simulink model "eCS_Algo_Simulation_2015b"  (R2015b)
settings: Solver=ode1  StartTime=0.0  StopTime=3  FixedStep=1/80000  RelTol=1e-3
PreLoadFcn:
  | if exist('tl_preloadfcn','file'), tl_preloadfcn(gcs,402); end
PostLoadFcn:
  | , if any(exist('dsrtsu_mdlpostloadfcn', 'file') == [2, 3, 6]), try dsrtsu_mdlpostloadfcn('Execute', bdroot); catch fprintf('Error in PostLoadFcn (dsrtsu_mdlpostloadfcn) for model "%s":\n %s\n', bdroot, lasterr); end, end,
  | if exist('tl_postloadfcn','file'), tl_postloadfcn(gcs,402); end
InitFcn:
  | Omegan=1.3024e+03;
  | xi=0.9; %0.48
  | K=0.1931;
  | K1=0.0198;
  | TauLocked=0.00255;
  | TauUnLocked=0.0042;
  | Kp=1/(2*K1);
  | Ki=Kp/((TauLocked+TauUnLocked)/2);
  | if exist('tlds_init','file'), tlds_init(gcs); end
StartFcn:
  | if exist('tlds_start','file'), tlds_start(gcs); end
StopFcn:
  | if exist('tlds_stop','file'), tlds_stop(gcs); end
model workspace (MAT data in the model file):
  au8PrevExecProfile = [0 0 0 0 0 0]
values from neighbouring files (symbols this model uses):
  AccSensor = 5    [Parameter_eCS_Algo.m]
  AlgoType = 0    [Parameter_eCS_Algo.m]
  Cxy = 1*0.017    (= 0.017)    [Acc_Init_SelV1.m]
  Cxz = 1*0.017    (= 0.017)    [Acc_Init_SelV1.m]
  Cyx = 1*0.017    (= 0.017)    [Acc_Init_SelV1.m]
  Cyz = 1*0.017    (= 0.017)    [Acc_Init_SelV1.m]
  Czx = 1*0.017    (= 0.017)    [Acc_Init_SelV1.m]
  Czy = 1*0.017    (= 0.017)    [Acc_Init_SelV1.m]
  Forced_Oscillation = 0    [Parameter_eCS_Algo.m]    (also in run_Rotation_sim.m = run)
  FreqTemperature = 10    [Acc_Init_SelV1.m]
  MaxSensorOffset = 0.3    [Acc_Init_SelV1.m]
  Mean_x_noise = 4e-3    (= 0.004)    [Acc_Init_SelV1.m]
  Mean_y_noise = 4e-3    (= 0.004)    [Acc_Init_SelV1.m]
  Mean_z_noise = 4e-3    (= 0.004)    [Acc_Init_SelV1.m]
  ODR = 8000    [Acc_Init_SelV1.m]
  offsetcorrection_on_off = 0    [Parameter_eCS_Algo.m]
  phi_pulse_rotation = 0    [Parameter_eCS_Algo.m]    (also in run_Rotation_sim.m = angle)
  pulsetype = 2    [Parameter_eCS_Algo.m]    (also in run_simulation.m = j; run_simulation_ActiveX.m = j)
  Range = 4    [Acc_Init_SelV1.m]
  sensitivity_optimisation = 0    [Parameter_eCS_Algo.m]
  TempBias = 0    [Acc_Init_SelV1.m]
  TemperatureAmp = 0    [Acc_Init_SelV1.m]
  Var_x_noise = 1.84e-9    (= 1.84e-09)    [Acc_Init_SelV1.m]
  Var_y_noise = 2.025e-09    [Acc_Init_SelV1.m]
  Var_z_noise = 1.374e-09    [Acc_Init_SelV1.m]
  w_x = 2*pi*F_x    (= 376.991118431)    [Acc_Init_SelV1.m]
  w_y = 2*pi*F_y    (= 376.991118431)    [Acc_Init_SelV1.m]
  w_z = 2*pi*F_z    (= 376.991118431)    [Acc_Init_SelV1.m]
  x_max_temp_drift = 0.061    [Acc_Init_SelV1.m]
  x_offset_enable = 0    [Acc_Init_SelV1.m]
  x_run_to_run_drift = 0.0    (= 0)    [Acc_Init_SelV1.m]
  x_temp_co_drift = 0.000    (= 0)    [Acc_Init_SelV1.m]
  Xi_x = 0.7    [Acc_Init_SelV1.m]
  Xi_y = 0.7    [Acc_Init_SelV1.m]
  Xi_z = 0.7    [Acc_Init_SelV1.m]
  y_max_temp_drift = 0.061    [Acc_Init_SelV1.m]
  y_offset_enable = 0    [Acc_Init_SelV1.m]
  y_run_to_run_drift = 0.0    (= 0)    [Acc_Init_SelV1.m]
  y_temp_co_drift = 0.000    (= 0)    [Acc_Init_SelV1.m]
  z_max_temp_drift = 0.13    [Acc_Init_SelV1.m]
  z_offset_enable = 0    [Acc_Init_SelV1.m]
  z_run_to_run_drift = 0.0    (= 0)    [Acc_Init_SelV1.m]
  z_temp_co_drift = 0.000    (= 0)    [Acc_Init_SelV1.m]
undefined symbols (not defined in the file or in its folder): controller_sample_rate, ddv, DiscIntNeverNeededParam, gmw_roada_x__m_s__, gmw_roada_y__m_s__, gmw_roadtime_2kHz, KSF_50_a_x, KSF_50_a_y, KSF_50_time, KSG_30_a_x, KSG_30_a_y, KSG_30_time, Meldorf_HindenburgstraAcceleration_x__m_s_2_, Meldorf_HindenburgstraAcceleration_y__m_s_2_, Meldorf_HindenburgstraAcceleration_z__m_s_2_, Meldorf_HindenburgstraTime__s_, pulse_FF27, pulse_MPDB, pulse_ODB40, pulse_ODB64, pulse_USNCAP, pulsetime_FF27, pulsetime_MPDB, pulsetime_ODB40, pulsetime_ODB64, pulsetime_USNCAP, Rauasphalt_60_a_x, Rauasphalt_60_a_y, Rauasphalt_60_time, sigbuilder_block, VW_416_2kHza_x_2kHz, VW_416_2kHza_y_2kHz, VW_416_2kHztime_2kHz
libraries: simulink x29, tllib x23, tl_autosar_lib x15, simulink_extras x7, LIB_TF_G_111 x2, LIB_TF_G_12_StepControl x2, LIB_TF_G_112 x1, dspsigops x1
(part 7 of 13)

== system eCS_Algo_Simulation_2015b/eCS/Subsystem/eCS/eCS/eCS_runMainFunction/BallAlgo ==
  note: [-1 : 1]
  note: [-25 ; 25]
  note: [-25 ;25]
  Pulses(x,y) : Inport
  b8IsSensitivityOpt : Inport  Port=2
  Add : Sum  Inputs=+--  mask(TL_Sum){data={'output',{'type','Int32','scaling','MperSecSqd_Algo/scIntegV_SI','show',1},'date',738573.71918759262}}
      settings: CopyFcn=if exist('tl_reset_reviewflag','file')==2,tl_reset_reviewflag(gcbh);end  DeleteFcn=if exist('delete_tlblock','file')==2,delete_tlblock(gcbh);end  NameChangeFcn=if exist('rename_tlblock','file')==2,rename_tlblock(gcbh);end  OpenFcn=if exist('tl_open_blockdlg','file')==2,tl_open_blockdlg(gcbh);else,open_system(gcbh,'parameter');end
      mask Help: eval(['if exist(''tl_online_help'',''file'') == 2, tl_online_help(''Topic'',''TL_Sum''),else, web([''jar:file:///'',matlabroot,''/help/toolbox/simulink/help.jar!/slref/' lower(get_param(gcbh,'Blocktype')) '.html''], ''-helpbrowser''),end'])
      mask Display: plot([-0.1, 1.05, NaN, -0.1, 1.05],[.01, .01, NaN, .99, .99]);
  Angle : Sum  mask(TL_Sum){data={'output',{'scaling','PowerOf2/scAngle','show',1},'date',738573.7191878357}}
      settings: AttributesFormatString=[Int16 2^-10]\n  CopyFcn=if exist('tl_reset_reviewflag','file')==2,tl_reset_reviewflag(gcbh);end  DeleteFcn=if exist('delete_tlblock','file')==2,delete_tlblock(gcbh);end  NameChangeFcn=if exist('rename_tlblock','file')==2,rename_tlblock(gcbh);end  OpenFcn=if exist('tl_open_blockdlg','file')==2,tl_open_blockdlg(gcbh);else,open_system(gcbh,'parameter');end
      mask Help: eval(['if exist(''tl_online_help'',''file'') == 2, tl_online_help(''Topic'',''TL_Sum''),else, web([''jar:file:///'',matlabroot,''/help/toolbox/simulink/help.jar!/slref/' lower(get_param(gcbh,'Blocktype')) '.html''], ''-helpbrowser''),end'])
      mask Display: plot([-0.1, 1.05, NaN, -0.1, 1.05],[.01, .01, NaN, .99, .99]);
  BallDamperSat : Saturate  UpperLimit=ddv('eCS_CFG/SI_Algo/BALL_DAMPER_SAT_MAX')  LowerLimit=ddv('eCS_CFG/SI_Algo/BALL_DAMPER_SAT_MIN')  mask(TL_Saturate){data={'output',{'type','Int32','scaling','MperSecSqd_Algo/scIntegV_SI','show',1},'lowerlimit',{'variable','eCS_CFG/SI_Algo/BALL_DAMPER_SAT_MIN'},'upperlimit',{'variable','eCS_CFG/SI_Algo/BALL_DAMPER_SAT_MAX'},'date',738573.7191880903}}
      settings: AttributesFormatString=[Int32 2^-16]\n  CopyFcn=if exist('tl_reset_reviewflag','file')==2,tl_reset_reviewflag(gcbh);end  DeleteFcn=if exist('delete_tlblock','file')==2,delete_tlblock(gcbh);end  NameChangeFcn=if exist('rename_tlblock','file')==2,rename_tlblock(gcbh);end  OpenFcn=if exist('tl_open_blockdlg','file')==2,tl_open_blockdlg(gcbh);else,open_system(gcbh,'parameter');end
      mask Help: eval(['if exist(''tl_online_help'',''file'') == 2, tl_online_help(''Topic'',''TL_Saturate''),else, web([''jar:file:///'',matlabroot,''/help/toolbox/simulink/help.jar!/slref/' lower(get_param(gcbh,'Blocktype')) '.html''], ''-helpbrowser''),end'])
      mask Display: plot([-0.1, 1.05, NaN, -0.1, 1.05],[.01, .01, NaN, .99, .99]);
  CalotteAngle1 : Gain  Gain=ddv('eCS_CFG/SI_Algo/S16_CALOTTE_ANGLE_1')  mask(TL_Gain){data={'output',{'scaling','PowerOf2/scAngle','show',1},'gain',{'variable','eCS_CFG/SI_Algo/S16_CALOTTE_ANGLE_1'},'date',738573.71918843745}}
      settings: AttributesFormatString=[Int16 2^-10]\n  CopyFcn=if exist('tl_reset_reviewflag','file')==2,tl_reset_reviewflag(gcbh);end  DeleteFcn=if exist('delete_tlblock','file')==2,delete_tlblock(gcbh);end  NameChangeFcn=if exist('rename_tlblock','file')==2,rename_tlblock(gcbh);end  OpenFcn=if exist('tl_open_blockdlg','file')==2,tl_open_blockdlg(gcbh);else,open_system(gcbh,'parameter');end
      mask Help: eval(['if exist(''tl_online_help'',''file'') == 2, tl_online_help(''Topic'',''TL_Gain''),else, web([''jar:file:///'',matlabroot,''/help/toolbox/simulink/help.jar!/slref/' lower(get_param(gcbh,'Blocktype')) '.html''], ''-helpbrowser''),end'])
      mask Display: plot([0, .88, 0],[.05, .5, .93]);
  CalotteAngle2 : Gain  Gain=ddv('eCS_CFG/SI_Algo/S16_CALOTTE_ANGLE_2')  mask(TL_Gain){data={'output',{'scaling','PowerOf2/scAngle','show',1},'gain',{'variable','eCS_CFG/SI_Algo/S16_CALOTTE_ANGLE_2'},'date',738573.71918868052}}
      settings: AttributesFormatString=[Int16 2^-10]\n  CopyFcn=if exist('tl_reset_reviewflag','file')==2,tl_reset_reviewflag(gcbh);end  DeleteFcn=if exist('delete_tlblock','file')==2,delete_tlblock(gcbh);end  NameChangeFcn=if exist('rename_tlblock','file')==2,rename_tlblock(gcbh);end  OpenFcn=if exist('tl_open_blockdlg','file')==2,tl_open_blockdlg(gcbh);else,open_system(gcbh,'parameter');end
      mask Help: eval(['if exist(''tl_online_help'',''file'') == 2, tl_online_help(''Topic'',''TL_Gain''),else, web([''jar:file:///'',matlabroot,''/help/toolbox/simulink/help.jar!/slref/' lower(get_param(gcbh,'Blocktype')) '.html''], ''-helpbrowser''),end'])
      mask Display: plot([0, .88, 0],[.05, .5, .93]);
  Cartesian To Polar : Subsystem  TreatAsAtomicUnit=on
  Demux : Demux  Outputs=2
  Function : tllib/Function  data={'stepfunctionname','ComputeBallPosition','date',738070.65144287038}  displayString=FUNCTION
  IntegSx : DiscreteIntegrator  SampleTime=-1  LimitOutput=on  UpperSaturationLimit=ddv('eCS_CFG/SI_Algo/BALL_POS_MAX')  LowerSaturationLimit=ddv('eCS_CFG/SI_Algo/BALL_POS_MIN')  ICPrevOutput=DiscIntNeverNeededParam  ICPrevScaledInput=DiscIntNeverNeededParam  mask(TL_DiscreteIntegrator){data={'logdata',{'loggingmode',1},'output',{'name','$D','scaling','MperSecSqd_Algo/scIntegS_SI','show',1},'state',{'scaling','MperSecSqd_Algo/scIntegS_SI'},'lowerlimit',{'variable','eCS_CFG/SI_Algo/BALL_POS_MIN'},'upperlimit',{'variable','eCS_CFG/SI_Algo/BALL_POS_MAX'},'date',738573.71919074073}}
      settings: AttributesFormatString=[Int16 2^-24]\n  CopyFcn=if exist('tl_reset_reviewflag') == 2, tl_reset_reviewflag(gcbh); end  DeleteFcn=if exist('delete_tlblock','file')==2,delete_tlblock(gcbh);end  NameChangeFcn=if exist('rename_tlblock','file')==2,rename_tlblock(gcbh);end  OpenFcn=if exist('tl_open_blockdlg','file')==2,tl_open_blockdlg(gcbh);else,open_system(gcbh,'parameter');end
      mask Help: eval(['if exist(''tl_online_help'',''file'') == 2, tl_online_help(''Topic'',''TL_DiscreteIntegrator''),else, web([''jar:file:///'',matlabroot,''/help/toolbox/simulink/help.jar!/slref/' lower(get_param(gcbh,'Blocktype')) '.html''], ''-helpbrowser''),end'])
      mask Display: plot([-0.1, 1.05, NaN, -0.1, 1.05],[.01, .01, NaN, .99, .99]);
  IntegSy : DiscreteIntegrator  SampleTime=-1  LimitOutput=on  UpperSaturationLimit=ddv('eCS_CFG/SI_Algo/BALL_POS_MAX')  LowerSaturationLimit=ddv('eCS_CFG/SI_Algo/BALL_POS_MIN')  ICPrevOutput=DiscIntNeverNeededParam  ICPrevScaledInput=DiscIntNeverNeededParam  mask(TL_DiscreteIntegrator){data={'logdata',{'loggingmode',1},'output',{'name','$D','scaling','MperSecSqd_Algo/scIntegS_SI','show',1},'state',{'scaling','MperSecSqd_Algo/scIntegS_SI'},'lowerlimit',{'variable','eCS_CFG/SI_Algo/BALL_POS_MIN'},'upperlimit',{'variable','eCS_CFG/SI_Algo/BALL_POS_MAX'},'date',738573.71919109952}}
      settings: AttributesFormatString=[Int16 2^-24]\n  CopyFcn=if exist('tl_reset_reviewflag') == 2, tl_reset_reviewflag(gcbh); end  DeleteFcn=if exist('delete_tlblock','file')==2,delete_tlblock(gcbh);end  NameChangeFcn=if exist('rename_tlblock','file')==2,rename_tlblock(gcbh);end  OpenFcn=if exist('tl_open_blockdlg','file')==2,tl_open_blockdlg(gcbh);else,open_system(gcbh,'parameter');end
      mask Help: eval(['if exist(''tl_online_help'',''file'') == 2, tl_online_help(''Topic'',''TL_DiscreteIntegrator''),else, web([''jar:file:///'',matlabroot,''/help/toolbox/simulink/help.jar!/slref/' lower(get_param(gcbh,'Blocktype')) '.html''], ''-helpbrowser''),end'])
      mask Display: plot([-0.1, 1.05, NaN, -0.1, 1.05],[.01, .01, NaN, .99, .99]);
  IntegVx : DiscreteIntegrator  SampleTime=-1  ICPrevOutput=DiscIntNeverNeededParam  ICPrevScaledInput=DiscIntNeverNeededParam  mask(TL_DiscreteIntegrator){data={'logdata',{'loggingmode',1},'output',{'scaling','MperSecSqd_Algo/scIntegV_SI','show',1},'state',{'scaling','MperSecSqd_Algo/scIntegV_SI'},'date',738573.71919129626}}
      settings: AttributesFormatString=[Int16 2^-16]\n  CopyFcn=if exist('tl_reset_reviewflag') == 2, tl_reset_reviewflag(gcbh); end  DeleteFcn=if exist('delete_tlblock','file')==2,delete_tlblock(gcbh);end  NameChangeFcn=if exist('rename_tlblock','file')==2,rename_tlblock(gcbh);end  OpenFcn=if exist('tl_open_blockdlg','file')==2,tl_open_blockdlg(gcbh);else,open_system(gcbh,'parameter');end
      mask Help: eval(['if exist(''tl_online_help'',''file'') == 2, tl_online_help(''Topic'',''TL_DiscreteIntegrator''),else, web([''jar:file:///'',matlabroot,''/help/toolbox/simulink/help.jar!/slref/' lower(get_param(gcbh,'Blocktype')) '.html''], ''-helpbrowser''),end'])
      mask Display: plot([-0.1, 1.05, NaN, -0.1, 1.05],[.01, .01, NaN, .99, .99]);
  IntegVy : DiscreteIntegrator  SampleTime=-1  ICPrevOutput=DiscIntNeverNeededParam  ICPrevScaledInput=DiscIntNeverNeededParam  mask(TL_DiscreteIntegrator){data={'output',{'scaling','MperSecSqd_Algo/scIntegV_SI','show',1},'state',{'scaling','MperSecSqd_Algo/scIntegV_SI'},'date',738573.71919152781}}
      settings: CopyFcn=if exist('tl_reset_reviewflag') == 2, tl_reset_reviewflag(gcbh); end  DeleteFcn=if exist('delete_tlblock','file')==2,delete_tlblock(gcbh);end  NameChangeFcn=if exist('rename_tlblock','file')==2,rename_tlblock(gcbh);end  OpenFcn=if exist('tl_open_blockdlg','file')==2,tl_open_blockdlg(gcbh);else,open_system(gcbh,'parameter');end
      mask Help: eval(['if exist(''tl_online_help'',''file'') == 2, tl_online_help(''Topic'',''TL_DiscreteIntegrator''),else, web([''jar:file:///'',matlabroot,''/help/toolbox/simulink/help.jar!/slref/' lower(get_param(gcbh,'Blocktype')) '.html''], ''-helpbrowser''),end'])
      mask Display: plot([-0.1, 1.05, NaN, -0.1, 1.05],[.01, .01, NaN, .99, .99]);
  Lut_Angle_1 : Lookup_n-D  NumberOfTableDimensions=1  BreakpointsForDimension1=ddv('eCS_CFG/SI_Algo/AU16_LUT_CALLOTE_ANGLE_1_IDX')  IndexSearchMethod=Linear search  Table=ddv('eCS_CFG/SI_Algo/AU16_LUT_CALLOTE_ANGLE_1_FACT')  ExtrapMethod=Clip  UseLastTableValue=on  InternalRulePriority=Speed  RndMeth=Simplest  InputSameDT=on  mask(TL_Lookup1D){data={'logdata',{'loggingmode',1},'input',{'variable','eCS_CFG/SI_Algo/AU16_LUT_CALLOTE_ANGLE_1_IDX'},'output',{'type','UInt16','scaling','PowerOf2/scLutY','show',1},'table',{'variable','eCS_CFG/SI_Algo/AU16_LUT_CALLOTE_ANGLE_1_FACT'},'map',{'name','CalotteAngle1_LUT','class','MERGEABLE_CONST'},'date',738573.71919193282}}
      settings: AttributesFormatString=[UInt16 2^-14]\n  CopyFcn=if exist('tl_reset_reviewflag','file')==2,tl_reset_reviewflag(gcbh);end  DeleteFcn=if exist('delete_tlblock','file')==2,delete_tlblock(gcbh);end  NameChangeFcn=if exist('rename_tlblock','file')==2,rename_tlblock(gcbh);end  OpenFcn=if exist('tl_open_blockdlg','file')==2,tl_open_blockdlg(gcbh);else,open_system(gcbh,'parameter');end
      mask Help: eval(['if exist(''tl_online_help'',''file'') == 2, tl_online_help(''Topic'',''TL_Lookup1D''),else, web([''jar:file:///'',matlabroot,''/help/toolbox/simulink/help.jar!/slref/' lower(get_param(gcbh,'Blocktype')) '.html''], ''-helpbrowser''),end'])
      mask Display: plot([-0.1, 1.05, NaN, -0.1, 1.05],[.01, .01, NaN, .99, .99]);
  Lut_Angle_2 : Lookup_n-D  NumberOfTableDimensions=1  BreakpointsForDimension1=ddv('eCS_CFG/SI_Algo/AU16_LUT_CALLOTE_ANGLE_2_IDX')  IndexSearchMethod=Linear search  Table=ddv('eCS_CFG/SI_Algo/AU16_LUT_CALLOTE_ANGLE_2_FACT')  ExtrapMethod=Clip  UseLastTableValue=on  InternalRulePriority=Speed  RndMeth=Simplest  InputSameDT=on  mask(TL_Lookup1D){data={'input',{'variable','eCS_CFG/SI_Algo/AU16_LUT_CALLOTE_ANGLE_2_IDX'},'output',{'scaling','PowerOf2/scLutY','show',1},'table',{'variable','eCS_CFG/SI_Algo/AU16_LUT_CALLOTE_ANGLE_2_FACT'},'map',{'name','CalotteAngle2_LUT','class','MERGEABLE_CONST'},'date',738573.71919232642}}
      settings: AttributesFormatString=[Int16 2^-14]\n  CopyFcn=if exist('tl_reset_reviewflag','file')==2,tl_reset_reviewflag(gcbh);end  DeleteFcn=if exist('delete_tlblock','file')==2,delete_tlblock(gcbh);end  NameChangeFcn=if exist('rename_tlblock','file')==2,rename_tlblock(gcbh);end  OpenFcn=if exist('tl_open_blockdlg','file')==2,tl_open_blockdlg(gcbh);else,open_system(gcbh,'parameter');end
      mask Help: eval(['if exist(''tl_online_help'',''file'') == 2, tl_online_help(''Topic'',''TL_Lookup1D''),else, web([''jar:file:///'',matlabroot,''/help/toolbox/simulink/help.jar!/slref/' lower(get_param(gcbh,'Blocktype')) '.html''], ''-helpbrowser''),end'])
      mask Display: plot([-0.1, 1.05, NaN, -0.1, 1.05],[.01, .01, NaN, .99, .99]);
  Mux : Mux  Inputs=2
  Mux1 : Mux  Inputs=2
  Product : Product  Inputs=**  RndMeth=Zero  mask(TL_Product){data={'output',{'scaling','MperSecSqd_Algo/scAccel_SI','show',1},'date',738573.71919256949}}
      settings: CopyFcn=if exist('tl_reset_reviewflag') == 2, tl_reset_reviewflag(gcbh); end  DeleteFcn=if exist('delete_tlblock','file')==2,delete_tlblock(gcbh);end  NameChangeFcn=if exist('rename_tlblock','file')==2,rename_tlblock(gcbh);end  OpenFcn=if exist('tl_open_blockdlg','file')==2,tl_open_blockdlg(gcbh);else,open_system(gcbh,'parameter');end
      mask Help: eval(['if exist(''tl_online_help'',''file'') == 2, tl_online_help(''Topic'',''TL_Product''),else, web([''jar:file:///'',matlabroot,''/help/toolbox/simulink/help.jar!/slref/' lower(get_param(gcbh,'Blocktype')) '.html''], ''-helpbrowser''),end'])
      mask Display: plot([-0.1, 1.05, NaN, -0.1, 1.05],[.01, .01, NaN, .99, .99]);
  Product1 : Product  Inputs=**  RndMeth=Zero  mask(TL_Product){data={'output',{'scaling','MperSecSqd_Algo/scAccel_SI','show',1},'date',738573.71919273143}}
      settings: CopyFcn=if exist('tl_reset_reviewflag') == 2, tl_reset_reviewflag(gcbh); end  DeleteFcn=if exist('delete_tlblock','file')==2,delete_tlblock(gcbh);end  NameChangeFcn=if exist('rename_tlblock','file')==2,rename_tlblock(gcbh);end  OpenFcn=if exist('tl_open_blockdlg','file')==2,tl_open_blockdlg(gcbh);else,open_system(gcbh,'parameter');end
      mask Help: eval(['if exist(''tl_online_help'',''file'') == 2, tl_online_help(''Topic'',''TL_Product''),else, web([''jar:file:///'',matlabroot,''/help/toolbox/simulink/help.jar!/slref/' lower(get_param(gcbh,'Blocktype')) '.html''], ''-helpbrowser''),end'])
      mask Display: plot([-0.1, 1.05, NaN, -0.1, 1.05],[.01, .01, NaN, .99, .99]);
  Relay : Relay  OnSwitchValue=ddv('eCS_CFG/SI_Algo/ECS_TRIGGER_ON')  OffSwitchValue=ddv('eCS_CFG/SI_Algo/ECS_TRIGGER_OFF')  mask(TL_Relay){data={'logdata',{'loggingmode',1},'output',{'type','Bool','unit','m','show',1},'onoutput',{'type','Bool','unit','m'},'offoutput',{'type','Bool','unit','m'},'onswitch',{'variable','eCS_CFG/SI_Algo/ECS_TRIGGER_ON'},'offswitch',{'variable','eCS_CFG/SI_Algo/ECS_TRIGGER_OFF'},'date',738573.71919327544}}
      settings: AttributesFormatString=[Bool ]\n  CopyFcn=if exist('tl_reset_reviewflag') == 2, tl_reset_reviewflag(gcbh); end  DeleteFcn=if exist('delete_tlblock','file')==2,delete_tlblock(gcbh);end  NameChangeFcn=if exist('rename_tlblock','file')==2,rename_tlblock(gcbh);end  OpenFcn=if exist('tl_open_blockdlg','file')==2,tl_open_blockdlg(gcbh);else,open_system(gcbh,'parameter');end
      mask Help: eval(['if exist(''tl_online_help'',''file'') == 2, tl_online_help(''Topic'',''TL_Relay''),else, web([''jar:file:///'',matlabroot,''/help/toolbox/simulink/help.jar!/slref/' lower(get_param(gcbh,'Blocktype')) '.html''], ''-helpbrowser''),end'])
      mask Display: plot([-0.1, 1.05, NaN, -0.1, 1.05],[.01, .01, NaN, .99, .99]);
  Sensitivity Optimization : Subsystem  TreatAsAtomicUnit=on
  Sin : Trigonometry  mask(TL_Trigonometry){data={'output',{'scaling','PowerOf2/scRadian','show',1},'date',738573.71919734951}}
      settings: CopyFcn=if exist('tl_reset_reviewflag','file')==2,tl_reset_reviewflag(gcbh);end  DeleteFcn=if exist('delete_tlblock','file')==2,delete_tlblock(gcbh);end  NameChangeFcn=if exist('rename_tlblock','file')==2,rename_tlblock(gcbh);end  OpenFcn=if exist('tl_open_blockdlg','file')==2,tl_open_blockdlg(gcbh);else,open_system(gcbh,'parameter');end
      mask Help: eval(['if exist(''tl_online_help'',''file'') == 2, tl_online_help(''Topic'',''TL_Trigonometry''),else, web([''jar:file:///'',matlabroot,''/help/toolbox/simulink/help.jar!/slref/' lower(get_param(gcbh,'Blocktype')) '.html''], ''-helpbrowser''),end'])
      mask Display: plot([-0.1, 1.05, NaN, -0.1, 1.05],[.01, .01, NaN, .99, .99]);
  ball damper : Gain  Gain=ddv('eCS_CFG/SI_Algo/BALL_DAMPER_COEFF')  mask(TL_Gain){data={'output',{'type','Int32','scaling','MperSecSqd_Algo/scIntegV_SI','show',1},'gain',{'variable','eCS_CFG/SI_Algo/BALL_DAMPER_COEFF'},'date',738573.71919762727}}
      settings: AttributesFormatString=[Int32 2^-16]\n  CopyFcn=if exist('tl_reset_reviewflag','file')==2,tl_reset_reviewflag(gcbh);end  DeleteFcn=if exist('delete_tlblock','file')==2,delete_tlblock(gcbh);end  NameChangeFcn=if exist('rename_tlblock','file')==2,rename_tlblock(gcbh);end  OpenFcn=if exist('tl_open_blockdlg','file')==2,tl_open_blockdlg(gcbh);else,open_system(gcbh,'parameter');end
      mask Help: eval(['if exist(''tl_online_help'',''file'') == 2, tl_online_help(''Topic'',''TL_Gain''),else, web([''jar:file:///'',matlabroot,''/help/toolbox/simulink/help.jar!/slref/' lower(get_param(gcbh,'Blocktype')) '.html''], ''-helpbrowser''),end'])
      mask Display: plot([0, .88, 0],[.05, .5, .93]);
  g to m.s² : Gain  Gain=9.807  mask(TL_Gain){data={'output',{'scaling','MperSecSqd_Algo/scAccel_SI','show',1},'date',738573.71919775463}}
      settings: AttributesFormatString=[Int16 2^-9]\n  CopyFcn=if exist('tl_reset_reviewflag','file')==2,tl_reset_reviewflag(gcbh);end  DeleteFcn=if exist('delete_tlblock','file')==2,delete_tlblock(gcbh);end  NameChangeFcn=if exist('rename_tlblock','file')==2,rename_tlblock(gcbh);end  OpenFcn=if exist('tl_open_blockdlg','file')==2,tl_open_blockdlg(gcbh);else,open_system(gcbh,'parameter');end
      mask Help: eval(['if exist(''tl_online_help'',''file'') == 2, tl_online_help(''Topic'',''TL_Gain''),else, web([''jar:file:///'',matlabroot,''/help/toolbox/simulink/help.jar!/slref/' lower(get_param(gcbh,'Blocktype')) '.html''], ''-helpbrowser''),end'])
      mask Display: plot([0, .88, 0],[.05, .5, .93]);
  grad in rad1 : Gain  Gain=pi/180  mask(TL_Gain){data={'output',{'scaling','PowerOf2/scLutY','show',1},'date',738573.71919800923}}
      settings: CopyFcn=if exist('tl_reset_reviewflag','file')==2,tl_reset_reviewflag(gcbh);end  DeleteFcn=if exist('delete_tlblock','file')==2,delete_tlblock(gcbh);end  NameChangeFcn=if exist('rename_tlblock','file')==2,rename_tlblock(gcbh);end  OpenFcn=if exist('tl_open_blockdlg','file')==2,tl_open_blockdlg(gcbh);else,open_system(gcbh,'parameter');end
      mask Help: eval(['if exist(''tl_online_help'',''file'') == 2, tl_online_help(''Topic'',''TL_Gain''),else, web([''jar:file:///'',matlabroot,''/help/toolbox/simulink/help.jar!/slref/' lower(get_param(gcbh,'Blocktype')) '.html''], ''-helpbrowser''),end'])
      mask Display: plot([0, .88, 0],[.05, .5, .93]);
  BallPosition(m) : Outport
  BallPosTrigger : Outport  Port=2
  wires:
  Sin/1 -> g to m.s²/1
  IntegVx/1 -> Mux1/1, IntegSx/1
  BallDamperSat/1 -> Add/3
  grad in rad1/1 -> Sin/1
  Lut_Angle_1/1 -> CalotteAngle1/1
  CalotteAngle1/1 -> Angle/1
  Lut_Angle_2/1 -> CalotteAngle2/1
  CalotteAngle2/1 -> Angle/2
  Angle/1 -> grad in rad1/1
  ball damper/1 -> BallDamperSat/1
  IntegSx/1 -> Cartesian To Polar/1(sBall_x)
  Cartesian To Polar/1(Radius_Sat) -> Lut_Angle_2/1, Relay/1, BallPosition(m)/1, Lut_Angle_1/1
  Cartesian To Polar/2(XFactor) -> [X_Factor]
  Cartesian To Polar/3(YFactor) -> [Y_Factor]
  [X_Factor] -> Product/1
  [Y_Factor] -> Product1/2
  g to m.s²/1 -> Product/2, Product1/1
  Mux/1 -> Add/2
  Product/1 -> Mux/1
  Product1/1 -> Mux/2
  Relay/1 -> BallPosTrigger/1
  Add/1 -> Demux/1  "a-ref"
  Demux/1 -> IntegVx/1
  Demux/2 -> IntegVy/1
  IntegVy/1 -> Mux1/2, IntegSy/1
  Mux1/1 -> ball damper/1
  IntegSy/1 -> Cartesian To Polar/2(sBall_y)
  Pulses(x,y)/1 -> Sensitivity Optimization/1(Pulse(x,y))
  Sensitivity Optimization/1(out_Pulse(x,y)) -> Add/1
  b8IsSensitivityOpt/1 -> Sensitivity Optimization/2(b8IsSensitivityOpt)

== system eCS_Algo_Simulation_2015b/eCS/Subsystem/eCS/eCS/eCS_runMainFunction/Crash Acceleration ==
  Ax : Inport
  Ay : Inport  Port=2
  Acceleration Clipping : Subsystem  TreatAsAtomicUnit=on
  Ax² : Product  Inputs=**  RndMeth=Zero  mask(TL_Product){data={'output',{'max',1538.84,'min',0,'type','UInt32','lsb',2^-18},'date',738573.71920496528}}
      settings: CopyFcn=if exist('tl_reset_reviewflag') == 2, tl_reset_reviewflag(gcbh); end  DeleteFcn=if exist('delete_tlblock','file')==2,delete_tlblock(gcbh);end  NameChangeFcn=if exist('rename_tlblock','file')==2,rename_tlblock(gcbh);end  OpenFcn=if exist('tl_open_blockdlg','file')==2,tl_open_blockdlg(gcbh);else,open_system(gcbh,'parameter');end
      mask Help: eval(['if exist(''tl_online_help'',''file'') == 2, tl_online_help(''Topic'',''TL_Product''),else, web([''jar:file:///'',matlabroot,''/help/toolbox/simulink/help.jar!/slref/' lower(get_param(gcbh,'Blocktype')) '.html''], ''-helpbrowser''),end'])
      mask Display: plot([-0.1, 1.05, NaN, -0.1, 1.05],[.01, .01, NaN, .99, .99]);
  Ax²Ay²Norm : Sqrt  SaturateOnIntegerOverflow=on  mask(TL_Sqrt){data={'output',{'type','UInt16','scaling','MperSecSqd_Algo/scAccel_SI'},'date',738573.71920506947}}
      settings: CopyFcn=if exist('tl_reset_reviewflag') == 2, tl_reset_reviewflag(gcbh); end  DeleteFcn=if exist('delete_tlblock','file')==2,delete_tlblock(gcbh);end  NameChangeFcn=if exist('rename_tlblock','file')==2,rename_tlblock(gcbh);end  OpenFcn=if exist('tl_open_blockdlg','file')==2,tl_open_blockdlg(gcbh);else,open_system(gcbh,'parameter');end
      mask Help: eval(['if exist(''tl_online_help'',''file'') == 2, tl_online_help(''Topic'',''TL_Sqrt''),else, web([''jar:file:///'',matlabroot,''/help/toolbox/simulink/help.jar!/slref/' lower(get_param(gcbh,'Blocktype')) '.html''], ''-helpbrowser''),end'])
      mask Display: plot([-0.1, 1.05, NaN, -0.1, 1.05],[.01, .01, NaN, .99, .99]);
  Ay² : Product  Inputs=**  RndMeth=Zero  mask(TL_Product){data={'output',{'max',1538.84,'min',0,'type','UInt32','lsb',2^-18},'date',738573.71920518519}}
      settings: CopyFcn=if exist('tl_reset_reviewflag') == 2, tl_reset_reviewflag(gcbh); end  DeleteFcn=if exist('delete_tlblock','file')==2,delete_tlblock(gcbh);end  NameChangeFcn=if exist('rename_tlblock','file')==2,rename_tlblock(gcbh);end  OpenFcn=if exist('tl_open_blockdlg','file')==2,tl_open_blockdlg(gcbh);else,open_system(gcbh,'parameter');end
      mask Help: eval(['if exist(''tl_online_help'',''file'') == 2, tl_online_help(''Topic'',''TL_Product''),else, web([''jar:file:///'',matlabroot,''/help/toolbox/simulink/help.jar!/slref/' lower(get_param(gcbh,'Blocktype')) '.html''], ''-helpbrowser''),end'])
      mask Display: plot([-0.1, 1.05, NaN, -0.1, 1.05],[.01, .01, NaN, .99, .99]);
  Function : tllib/Function  data={'stepfunctionname','CrashDetectionMtrPerSecSqd','date',737961.39265859954}  displayString=FUNCTION
  Sum : Sum  mask(TL_Sum){data={'output',{'type','UInt32','lsb',2^-18},'date',738573.71920542826}}
      settings: CopyFcn=if exist('tl_reset_reviewflag') == 2, tl_reset_reviewflag(gcbh); end  DeleteFcn=if exist('delete_tlblock','file')==2,delete_tlblock(gcbh);end  NameChangeFcn=if exist('rename_tlblock','file')==2,rename_tlblock(gcbh);end  OpenFcn=if exist('tl_open_blockdlg','file')==2,tl_open_blockdlg(gcbh);else,open_system(gcbh,'parameter');end
      mask Help: eval(['if exist(''tl_online_help'',''file'') == 2, tl_online_help(''Topic'',''TL_Sum''),else, web([''jar:file:///'',matlabroot,''/help/toolbox/simulink/help.jar!/slref/' lower(get_param(gcbh,'Blocktype')) '.html''], ''-helpbrowser''),end'])
      mask Display: plot([-0.1, 1.05, NaN, -0.1, 1.05],[.01, .01, NaN, .99, .99]);
  b8CrashTrigger : Outport
  wires:
  Sum/1 -> Ax²Ay²Norm/1
  Ay²/1 -> Sum/2
  Ax²/1 -> Sum/1
  Ax/1 -> Ax²/1, Ax²/2
  Ay/1 -> Ay²/2, Ay²/1
  Ax²Ay²Norm/1 -> Acceleration Clipping/1(u16AccelNorm)
  Acceleration Clipping/1(u8Trigger) -> b8CrashTrigger/1
